simulink model "sim_localization"  (R2025b)
settings: Solver=ode4  StartTime=0.0  StopTime=10.0  FixedStep=1e-3  RelTol=1e-3
values from neighbouring files (symbols this model uses):
  d_actual = 0.164    [init_localization.m]
  PHI_INIT = [0;0]    [id.m]    (also in init_localization.m)
  Q_INIT = q(:,1)    [id.m]    (also in init_localization.m)
  r_actual = 0.031    [init_localization.m]
  T_s = 0.04    [id.m]    (also in init_localization.m = 0.001)
settings Model: Creator=llp  LastModifiedBy=llp

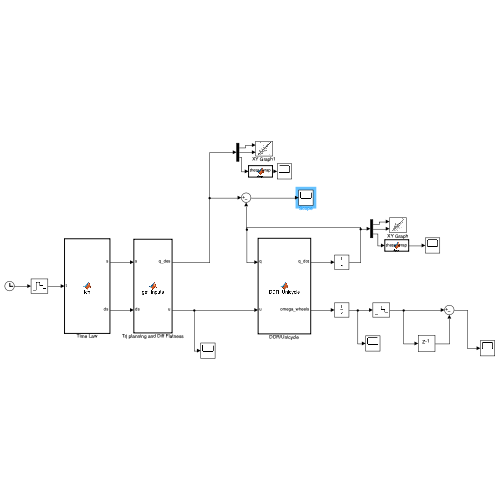
[thumbnail: Simulink's stored preview of the top-level diagram]
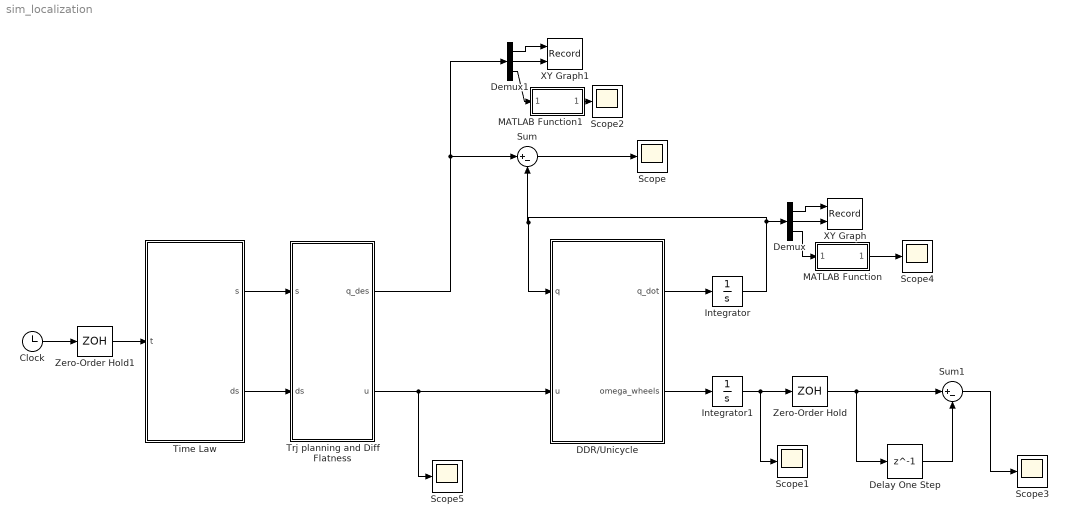
== system sim_localization ==
  Clock : Clock
  DDR/Unicycle : MATLAB Function  TreatAsAtomicUnit=on
  Delay One Step : Delay  DelayLength=1  SampleTime=T_s
  Demux : Demux  Outputs=3
  Demux1 : Demux  Outputs=3
  Integrator : Integrator  InitialCondition=Q_INIT
  Integrator1 : Integrator  InitialCondition=PHI_INIT
  MATLAB Function : MATLAB Function  TreatAsAtomicUnit=on
  MATLAB Function1 : MATLAB Function  TreatAsAtomicUnit=on
  Scope{,1..5} (6 alike) : Scope
      Scope settings: ActiveDisplayYMinimum=-7.1641531907927  ActiveDisplayYMaximum=0.8819382189103091
      Scope2 settings: ActiveDisplayYMinimum=-1  ActiveDisplayYMaximum=1  DataLoggingVariableName=ScopeData2
      Scope3 settings: ActiveDisplayYMinimum=-1  ActiveDisplayYMaximum=1  DataLoggingVariableName=ScopeData3
      Scope4 settings: ActiveDisplayYMinimum=-1  ActiveDisplayYMaximum=1  DataLoggingVariableName=ScopeData4
      Scope5 settings: ActiveDisplayYMinimum=-4.8188088205443105  ActiveDisplayYMaximum=4.8188088205443105  DataLoggingVariableName=ScopeData5
  Sum : Sum  Inputs=|+-
  Sum1 : Sum  Inputs=|+-
  Time Law : MATLAB Function  TreatAsAtomicUnit=on
  Trj planning and Diff Flatness : MATLAB Function  TreatAsAtomicUnit=on
  XY Graph : Record  NumPorts=2.0  FileSettingsInternal="{\"entries\":[{\"content\":{\"excelSettings\":{\"content\":{},\"type\":\"Streamout.ExcelSettings\"},\"parquetSettings\":{\"content\":{},\"type\":\"Streamout.ParquetSettings\"}},\"type\":\"Streamout.FileSettingStorage\",\"uuid\":\"\"}],\"packageUris\":[\"http:\\/\\/schema.mathworks.com\\/mf0\\/streamout_blocks\\/R2020a\"],\"version\":\"1.0\"}"  FrameSettings=[0, 0]  Layout=[1 1]  SignalsInternal="{\"entries\":[{\"content\":{\"signals\":[{\"content\":{\"blockPath\":[],\"dimensions\":[1,1],\"domain\":\"\",\"lineColor\":\"#a2142f\",\"plots\":[ 1 ],\"port\":1,\"sid\":[\"\"],\"signalID\":1,\"signalName\":\"Demux:1\"},\"type\":\"RecordBlkView.Signal\",\"uuid\":\"\"},{\"content\":{\"blockPath\":[],\"dimensions\":[1,1],\"domain\":\"\",\"lineColor\":\"#139fff\",\"plots\":[ 1 ],\"port\":2,\"sid\":[\"\"],\"signalID\":2,\"signalName\":\"Demux:2\"},\"type\":\"RecordBlkView.Signal\",\"uuid\":\"\"}]},\"type\":\"RecordBlkView.InputSignals\",\"uuid\":\"\"}],\"packageUris\":[\"http:\\/\\/schema.mathworks.com\\/mf0\\/streamout_blocks\\/R2020a\"],\"version\":\"1.0\"}"  VisualizationBindings="{\"xyplotplugin\":{\"info\":[{\"series\":[{\"bindingParametersList\":[{\"parameter\":\"X-Axis\",\"signalID\":1,\"signalName\":\"Demux:1\"},{\"parameter\":\"Y-Axis\",\"signalID\":2,\"signalName\":\"Demux:2\"}],\"seriesID\":0}],\"subplotID\":1}]}}"  CompatibilityTag=XY
  XY Graph1 : Record  NumPorts=2.0  FileSettingsInternal="{\"entries\":[{\"content\":{\"excelSettings\":{\"content\":{},\"type\":\"Streamout.ExcelSettings\"},\"parquetSettings\":{\"content\":{},\"type\":\"Streamout.ParquetSettings\"}},\"type\":\"Streamout.FileSettingStorage\",\"uuid\":\"\"}],\"packageUris\":[\"http:\\/\\/schema.mathworks.com\\/mf0\\/streamout_blocks\\/R2020a\"],\"version\":\"1.0\"}"  FrameSettings=[0, 0]  Layout=[1 1]  SignalsInternal="{\"entries\":[{\"content\":{\"signals\":[{\"content\":{\"blockPath\":[],\"dimensions\":[1,1],\"domain\":\"\",\"lineColor\":\"#a2142f\",\"plots\":[ 1 ],\"port\":1,\"sid\":[\"\"],\"signalID\":1,\"signalName\":\"Demux1:1\"},\"type\":\"RecordBlkView.Signal\",\"uuid\":\"\"},{\"content\":{\"blockPath\":[],\"dimensions\":[1,1],\"domain\":\"\",\"lineColor\":\"#139fff\",\"plots\":[ 1 ],\"port\":2,\"sid\":[\"\"],\"signalID\":2,\"signalName\":\"Demux1:2\"},\"type\":\"RecordBlkView.Signal\",\"uuid\":\"\"}]},\"type\":\"RecordBlkView.InputSignals\",\"uuid\":\"\"}],\"packageUris\":[\"http:\\/\\/schema.mathworks.com\\/mf0\\/streamout_blocks\\/R2020a\"],\"version\":\"1.0\"}"  VisualizationBindings="{\"xyplotplugin\":{\"info\":[{\"series\":[{\"bindingParametersList\":[{\"parameter\":\"X-Axis\",\"signalID\":1,\"signalName\":\"Demux1:1\"},{\"parameter\":\"Y-Axis\",\"signalID\":2,\"signalName\":\"Demux1:2\"}],\"seriesID\":0}],\"subplotID\":1}]}}"  CompatibilityTag=XY
  Zero-Order Hold : ZeroOrderHold  SampleTime=T_s
  Zero-Order Hold1 : ZeroOrderHold  SampleTime=T_s
  wires:
  Clock/1 -> Zero-Order Hold1/1
  Time Law/1(s) -> Trj planning and Diff Flatness/1(s)
  Time Law/2(ds) -> Trj planning and Diff Flatness/2(ds)
  DDR/Unicycle/1(q_dot) -> Integrator/1
  Trj planning and Diff Flatness/2(u) -> Scope5/1, DDR/Unicycle/2(u)
  Integrator/1 -> Demux/1, Sum/2, DDR/Unicycle/1(q)
  Trj planning and Diff Flatness/1(q_des) -> Demux1/1, Sum/1
  Sum/1 -> Scope/1
  DDR/Unicycle/2(omega_wheels) -> Integrator1/1
  Integrator1/1 -> Zero-Order Hold/1, Scope1/1
  Demux/1 -> XY Graph/1
  Demux/2 -> XY Graph/2
  Demux/3 -> MATLAB Function/1(theta)
  Demux1/2 -> XY Graph1/2
  Demux1/3 -> MATLAB Function1/1(theta)
  Demux1/1 -> XY Graph1/1
  MATLAB Function/1(wrap) -> Scope4/1
  MATLAB Function1/1(wrap) -> Scope2/1
  Zero-Order Hold/1 -> Delay One Step/1, Sum1/1
  Delay One Step/1 -> Sum1/2
  Sum1/1 -> Scope3/1
  Zero-Order Hold1/1 -> Time Law/1(t)

== matlab function sim_localization/Time Law ==
  data: t input; s output; ds output
function [s, ds] = fcn(t)
    
    Ta = 0.5;
    Tc = 9; 
        
    vc = 1/(Ta+Tc);
    a = vc/Ta;
   
    if t < Ta
        s_dot = a*t;
        s = 0.5*a*t^2;
    
    elseif t < (Ta+Tc)
        s_dot = vc;
        s = 0.5*a*Ta^2 + vc*(t - Ta);
    
    elseif t < (2*Ta+Tc)
        s_dot = vc - a*(t - Ta - Tc);
        s = 0.5*a*Ta^2 + vc*Tc + vc*(t - Ta - Tc) ...
            - 0.5*a*(t - Ta - Tc)^2;
    else
        s_dot = 0;
        s = 1;
    end

    ds = s_dot;
    
end

== matlab function sim_localization/DDR//Unicycle ==
  data: q input; u input; q_dot output; omega_wheels output; d_actual parameter; r_actual parameter
function [q_dot, omega_wheels] = DDR_Unicycle(q, u, d_actual, r_actual)

    % extract variables
    v = u(1);
    omega = u(2);

    q_dot= zeros(3,1);
    
    q_dot(1) = v*cos(q(3));
    q_dot(2) = v*sin(q(3));
    q_dot(3) = omega;

    
    wL = v/r_actual - d_actual/(2*r_actual) * omega;
    wR = v/r_actual + d_actual/(2*r_actual) * omega;

    omega_wheels = [wL; wR];

end

== matlab function sim_localization/Trj planning and Diff Flatness ==
  data: q_des output; s input; u output; ds input
function [q_des, u] = get_inputs(s, ds)

R = 0.4;
omega = 2*pi;

x = R*sin(2*omega*s);
y = R*sin(omega*s);

dx_ds = 2*omega*R*cos(2*omega*s);
dy_ds = omega*R*cos(omega*s);

ddx_ds2 = -4*omega^2*R*sin(2*omega*s);
ddy_ds2 = -omega^2*R*sin(omega*s);



theta = atan2(dy_ds, dx_ds);

q_des = [x; y; theta];

v = ds* sqrt(dx_ds^2 + dy_ds^2);

omega_input = ds* (dx_ds*ddy_ds2 - dy_ds*ddx_ds2) / (dx_ds^2 + dy_ds^2+10^-3);

u = [v; omega_input];

end

== matlab function sim_localization/MATLAB Function ==
  data: theta input; wrap output
function wrap = fcn(theta)

wrap = mod(theta+pi,2*pi)-pi ;

== matlab function sim_localization/MATLAB Function1 ==
  data: theta input; wrap output
function wrap = fcn(theta)

wrap = mod(theta+pi,2*pi)-pi ;
